simulink subsystem "balrobot_SubSystem"  (R2021a)
settings: Solver=VariableStepAuto  StartTime=0.0  StopTime=10.0  RelTol=1e-3
settings Model: Creator=umberto  LastModifiedBy=utente-A
settings SolverCC: AlgebraicLoopSolver=TrustRegion
settings DebuggingCC: SFMachineParentedDataDiag=warning

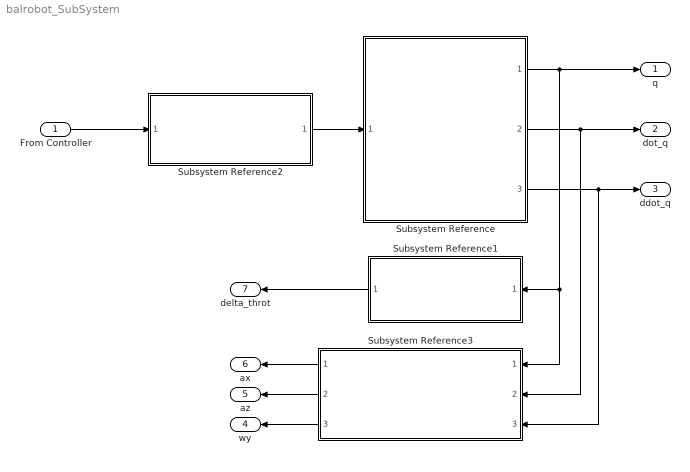
== system balrobot_SubSystem ==
  From Controller : Inport
  Subsystem Reference : Subsystem  ReferencedSubsystem=Electromechanical_SubSystem
  Subsystem Reference1 : Subsystem  ReferencedSubsystem=Encoder_SubSystem
  Subsystem Reference2 : Subsystem  ReferencedSubsystem=VoltageDriver_SubSystem
  Subsystem Reference3 : Subsystem  ReferencedSubsystem=MPU_SubSystem
  q : Outport
  dot_q : Outport  Port=2
  ddot_q : Outport  Port=3
  wy : Outport  Port=4
  az : Outport  Port=5
  ax : Outport  Port=6
  delta_throt : Outport  Port=7
  wires:
  Subsystem Reference2/1 -> Subsystem Reference/1
  Subsystem Reference/2 -> Subsystem Reference3/2, dot_q/1
  Subsystem Reference/3 -> Subsystem Reference3/3, ddot_q/1
  Subsystem Reference/1 -> Subsystem Reference3/1, Subsystem Reference1/1, q/1
  Subsystem Reference1/1 -> delta_throt/1
  Subsystem Reference3/1 -> ax/1
  From Controller/1 -> Subsystem Reference2/1
  Subsystem Reference3/2 -> az/1
  Subsystem Reference3/3 -> wy/1
